simulink model "PWM_and_Servo"  (Simulink 7.4)
settings: Solver=ode1  SolverMode=SingleTasking  StartTime=0.0  StopTime=inf  FixedStep=0.01  MaxStep=0.02  RelTol=1e-3  AbsTol=1e-6
undefined symbols (not defined in the file or in its folder): bit
libraries: mc9s12tool x3, simulink x1
CloseFcn:
  | rtwprivate ssgencode ModelCloseRequest MC_AD
settings Model: Creator=fwornle  LastModifiedBy=fw  SimulationMode=external  ExtModeTrigDuration=10000
settings ConfigSet: Description=rtmc9s12target_R2009b
settings DataIOCC: LimitDataPoints=off  SaveOutput=off  SaveTime=off  SignalLoggingName=sigsOut
settings OptimizationCC: BlockReduction=off  BooleanDataType=off  InitFltsAndDblsToZero=on  OptimizeModelRefInitCode=on  LifeSpan=1
settings DebuggingCC: SaveWithParameterizedLinksMsg=none  SignalResolutionControl=TryResolveAllWithWarning  SolverPrmCheckMsg=none  MultiTaskDSMMsg=warning  MultiTaskCondExecSysMsg=none  StrictBusMsg=None
settings HardwareCC: ProdBitPerInt=16  ProdEndianess=BigEndian  ProdWordSize=16  ProdHWDeviceType=Motorola HC12
settings RTWCC: SystemTargetFile=mc9s12.tlc  GenerateMakefile=off  TemplateMakefile=mc9s12.tmf  ProcessScript=mc9s12_make_rtw_hook  IncludeERTFirstTime=on
settings CodeAppCC: IgnoreCustomStorageClasses=off
settings STFCustomTargetCC: TargetFcnLib=ansi_tfl_tmw.mat  ModelReferenceCompliant=off  IncludeMdlTerminateFcn=off  ERTCustomFileBanners=on  SupportNonInlinedSFcns=off  CPPClassGenCompliant=on  SystemTargetFile=mc9s12.tlc
settings ERTTargetCC: TargetFcnLib=ansi_tfl_tmw.mat  MultiwordLength=2048  ModelReferenceCompliant=off  ParMdlRefBuildCompliant=off  CompOptLevelCompliant=off  IncludeMdlTerminateFcn=off  CombineOutputUpdateFcns=off  ERTFirstTimeCompliant=off  SupportContinuousTime=on  ModelStepFunctionPrototypeControlCompliant=off  ExtMode=on  ExtModeMexFile=ext_serial_mc9s12_comm  ExtModeMexArgs=1,2,115200  InlinedParameterPlacement=NonHierarchical  ERTCustomFileTemplate=mc9s12_file_process.tlc  GRTInterface=on  ConvertIfToSwitch=off
settings CustomProperty: DataType=RTWOptions_EnumType_C__Users_fw__SVN_rtmc9s12-target_trunk_rtmc9s12_CW_R2009b_bin_mc9s12_1mc9s12_TargetBoard  Value=Dragon12Plus
settings EnumStrPairs: String=Dragon12

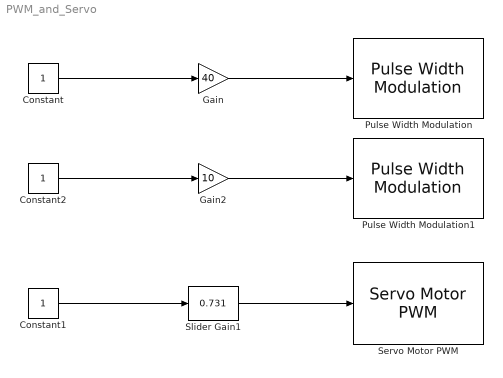
== system PWM_and_Servo ==
  Constant : Constant  OutDataType=sfix(16)  OutScaling=2^0
  Constant1 : Constant  OutDataType=sfix(16)  OutScaling=2^0
  Constant2 : Constant  OutDataType=sfix(16)  OutScaling=2^0
  Gain : Gain  Gain=40  ParameterDataType=sfix(16)  ParameterScaling=2^0  OutDataType=sfix(16)  OutScaling=2^0  SaturateOnIntegerOverflow=on  OutDataTypeStr=Inherit: Same as input  ParamDataTypeStr=Inherit: Same as input
  Gain2 : Gain  Gain=10  ParameterDataType=sfix(16)  ParameterScaling=2^0  OutDataType=sfix(16)  OutScaling=2^0  SaturateOnIntegerOverflow=on  OutDataTypeStr=Inherit: Same as input  ParamDataTypeStr=Inherit: Same as input
  Pulse Width Modulation : mc9s12tool/Pulse Width Modulation  Tag=mcTarget_pwm  SystemSampleTime=-1  sampletime=0.01  resolution=16 bit  PWMperiod=1  pulse_pin="1  (8-bit / 16-bit)"  sign_port=PTH  sign_pin=1  Vmax=100  sig_mon=off
  Pulse Width Modulation1 : mc9s12tool/Pulse Width Modulation  Tag=mcTarget_pwm  SystemSampleTime=-1  sampletime=0.01  resolution=16 bit  PWMperiod=0.5  pulse_pin="5  (8-bit / 16-bit)"  sign_port=PTH  sign_pin=2  Vmax=100  sig_mon=off
  Servo Motor PWM : mc9s12tool/Servo Motor PWM  Tag=mcTarget_pwmServo  SystemSampleTime=-1  sampletime=0.02  PWMperiod=0.02  minwidth=0.0006  maxwidth=0.0020  resolution=16 bit  pulse_pin="3  (8-bit / 16-bit)"  Vmax=1
  Slider Gain1 : simulink/Math Operations/Slider Gain  SystemSampleTime=-1  low=0  gain=0.731  high=1
  wires:
  Gain/1 -> Pulse Width Modulation/1
  Constant/1 -> Gain/1
  Gain2/1 -> Pulse Width Modulation1/1
  Constant2/1 -> Gain2/1
  Constant1/1 -> Slider Gain1/1
  Slider Gain1/1 -> Servo Motor PWM/1
